simulink model "my_model"  (R2018a)
settings: Solver=VariableStepAuto  StartTime=0.0  StopTime=50  RelTol=1e-3
values from neighbouring files (symbols this model uses):
  KT = 0.25    [DC_Motormfile.m]    (also in pid.m)
  L = 493*10^-9    (= 4.93e-07)    [DC_Motormfile.m]    (also in pid.m)
  R = 5.3*10^-3    (= 0.0053)    [DC_Motormfile.m]    (also in pid.m)
  Scaling_Velocity = Sc/(Cw)*Rg*KE    (= 4.865)    [pid.m]
  Ts = 0.01    [pid.m]
libraries: simulink x2
settings Model: Creator=MAFAZ  LastModifiedBy=MAFAZ

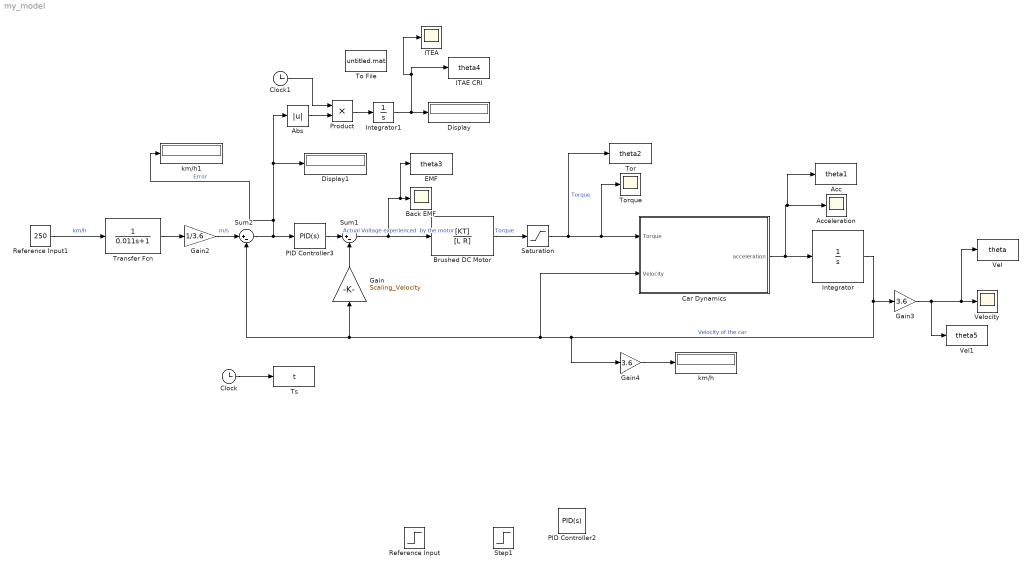
== system my_model ==
  Abs : Abs
  Acc : ToWorkspace  VariableName=theta1  SampleTime=Ts
  Acceleration : Scope
  Back EMF : Scope
  Brushed DC Motor : TransferFcn  Numerator=[KT]  Denominator=[L R]
  Car Dynamics : MATLAB Function  TreatAsAtomicUnit=on
  Clock : Clock
  Clock1 : Clock
  Display : Display
  Display1 : Display
  EMF : ToWorkspace  VariableName=theta3  SampleTime=Ts
  Gain : Gain  Gain=Scaling_Velocity
  Gain2 : Gain  Gain=1/3.6
  Gain3 : Gain  Gain=3.6
  Gain4 : Gain  Gain=3.6
  ITAE CRI : ToWorkspace  VariableName=theta4  SampleTime=Ts
  ITEA : Scope
  Integrator : Integrator
  Integrator1 : Integrator
  PID Controller2 : simulink/Continuous/PID Controller  Controller=PID  TimeDomain=Continuous-time  SampleTime=-1  IntegratorMethod=Forward Euler  FilterMethod=Forward Euler  Form=Parallel  UseFilter=on  ControllerParametersSource=internal  P=1.4  I=0.991  D=0  N=100  InitialConditionSource=internal  InitialConditionForIntegrator=0  InitialConditionForFilter=0  ExternalReset=none  LimitOutput=on  UpperSaturationLimit=346  LowerSaturationLimit=0  LinearizeAsGain=on  AntiWindupMode=none  Kb=1  TrackingMode=off  Kt=1  PParamMin=[]  PParamMax=[]  IParamMin=[]  IParamMax=[]  DParamMin=[]  DParamMax=[]  NParamMin=[]  NParamMax=[]  KbParamMin=[]  KbParamMax=[]  KtParamMin=[]  KtParamMax=[]  POutMin=[]  POutMax=[]  IOutMin=[]  IOutMax=[]  DOutMin=[]  DOutMax=[]  NOutMin=[]  NOutMax=[]  KbOutMin=[]  KbOutMax=[]  KtOutMin=[]  KtOutMax=[]  IntegratorOutMin=[]  IntegratorOutMax=[]  FilterOutMin=[]  FilterOutMax=[]  SumOutMin=[]  SumOutMax=[]  SumI1OutMin=[]  SumI1OutMax=[]  SumI2OutMin=[]  SumI2OutMax=[]  SumI3OutMin=[]  SumI3OutMax=[]  SumDOutMin=[]  SumDOutMax=[]  SaturationOutMin=[]  SaturationOutMax=[]  IntegratorContinuousStateAttributes=''  IntegratorStateMustResolveToSignalObject=off  IntegratorRTWStateStorageClass=Auto  FilterContinuousStateAttributes=''  FilterStateMustResolveToSignalObject=off  FilterRTWStateStorageClass=Auto  DifferentiatorICPrevScaledInput=0  DifferentiatorOutMin=[]  DifferentiatorOutMax=[]  FilterDiffOutCoefMin=[]  FilterDiffOutCoefMax=[]  SumDenOutMin=[]  SumDenOutMax=[]  SumNumOutMin=[]  SumNumOutMax=[]  ReciprocalOutMin=[]  ReciprocalOutMax=[]  DivideOutMin=[]  DivideOutMax=[]  TunerSelectOption=Transfer Function Based (PID Tuner App)
  PID Controller3 : simulink/Continuous/PID Controller  Controller=PID  TimeDomain=Continuous-time  SampleTime=-1  IntegratorMethod=Forward Euler  FilterMethod=Forward Euler  Form=Parallel  UseFilter=on  ControllerParametersSource=internal  P=9.2798502496609  I=30.752257407088  D=-0.724277837575087  N=6.32200896088574  InitialConditionSource=internal  InitialConditionForIntegrator=0  InitialConditionForFilter=0  ExternalReset=none  LimitOutput=on  UpperSaturationLimit=346  LowerSaturationLimit=0  LinearizeAsGain=on  AntiWindupMode=none  Kb=1  TrackingMode=off  Kt=1  PParamMin=[]  PParamMax=[]  IParamMin=[]  IParamMax=[]  DParamMin=[]  DParamMax=[]  NParamMin=[]  NParamMax=[]  KbParamMin=[]  KbParamMax=[]  KtParamMin=[]  KtParamMax=[]  POutMin=[]  POutMax=[]  IOutMin=[]  IOutMax=[]  DOutMin=[]  DOutMax=[]  NOutMin=[]  NOutMax=[]  KbOutMin=[]  KbOutMax=[]  KtOutMin=[]  KtOutMax=[]  IntegratorOutMin=[]  IntegratorOutMax=[]  FilterOutMin=[]  FilterOutMax=[]  SumOutMin=[]  SumOutMax=[]  SumI1OutMin=[]  SumI1OutMax=[]  SumI2OutMin=[]  SumI2OutMax=[]  SumI3OutMin=[]  SumI3OutMax=[]  SumDOutMin=[]  SumDOutMax=[]  SaturationOutMin=[]  SaturationOutMax=[]  IntegratorContinuousStateAttributes=''  IntegratorStateMustResolveToSignalObject=off  IntegratorRTWStateStorageClass=Auto  FilterContinuousStateAttributes=''  FilterStateMustResolveToSignalObject=off  FilterRTWStateStorageClass=Auto  DifferentiatorICPrevScaledInput=0  DifferentiatorOutMin=[]  DifferentiatorOutMax=[]  FilterDiffOutCoefMin=[]  FilterDiffOutCoefMax=[]  SumDenOutMin=[]  SumDenOutMax=[]  SumNumOutMin=[]  SumNumOutMax=[]  ReciprocalOutMin=[]  ReciprocalOutMax=[]  DivideOutMin=[]  DivideOutMax=[]  TunerSelectOption=Transfer Function Based (PID Tuner App)
  Product : Product
  Reference Input1 : Constant  Value=250
  "Reference Input " : Step  Time=0  After=346  SampleTime=0
  Saturation : Saturate  UpperLimit=600  LowerLimit=0
  Step1 : Step  Before=50  After=250  SampleTime=0
  Sum1 : Sum  Inputs=|+-
  Sum2 : Sum  Inputs=|+-
  To File : ToFile  SaveFormat=Timeseries
  Tor : ToWorkspace  VariableName=theta2  SampleTime=Ts
  Torque : Scope
  Transfer Fcn : TransferFcn  Denominator=[0.011 1]
  Ts : ToWorkspace  VariableName=t  SampleTime=Ts
  Vel : ToWorkspace  VariableName=theta  SampleTime=Ts
  Vel1 : ToWorkspace  VariableName=theta5  SampleTime=Ts
  Velocity : Scope
  km/h : Display
  km/h1 : Display
  wires:
  Gain/1 -> Sum1/2
  Sum1/1 -> EMF/1, Back EMF/1, Brushed DC Motor/1  "Actual Voltage experienced  by the motor"
  Brushed DC Motor/1 -> Saturation/1  "Torque"
  Saturation/1 -> Tor/1, Torque/1, Car Dynamics/1(Torque)  "Torque"
  Car Dynamics/1(acceleration) -> Acc/1, Acceleration/1, Integrator/1
  Integrator/1 -> Gain3/1, Gain4/1, Car Dynamics/2(Velocity), Sum2/2, Gain/1  "Velocity of the car"
  Clock/1 -> Ts/1
  Reference Input1/1 -> Transfer Fcn/1  "km/h"
  PID Controller3/1 -> Sum1/1
  Gain2/1 -> Sum2/1  "m/s"
  Sum2/1 -> PID Controller3/1, km/h1/1, Display1/1, Abs/1  "Error"
  Gain4/1 -> km/h/1
  Product/1 -> Integrator1/1
  Integrator1/1 -> ITEA/1, ITAE CRI/1, Display/1
  Abs/1 -> Product/2
  Clock1/1 -> Product/1
  Gain3/1 -> Vel1/1, Vel/1, Velocity/1
  Transfer Fcn/1 -> Gain2/1

== matlab function my_model/Car Dynamics ==
  data: Torque input; acceleration output; Velocity input
function acceleration = fcn(Torque, Velocity)
acceleration = (40.5*Torque*0.6-413-0.3381*Velocity^2)/2108;

% 0.6 = mechanical efficiency of the vehcile - to ensure its reaches 100
% km/h within 4.4 secs. 

% 413 = actual Rolling Resistance 
%0.3381 = drag force created by the movement of the car

%2108 = mass of the car
